simulink model "pv_model"  (R2023b)
settings: Solver=VariableStepAuto  StartTime=0.0  StopTime=10.0  RelTol=1e-3
libraries: simulink x1
settings Model: Creator=User  LastModifiedBy=User

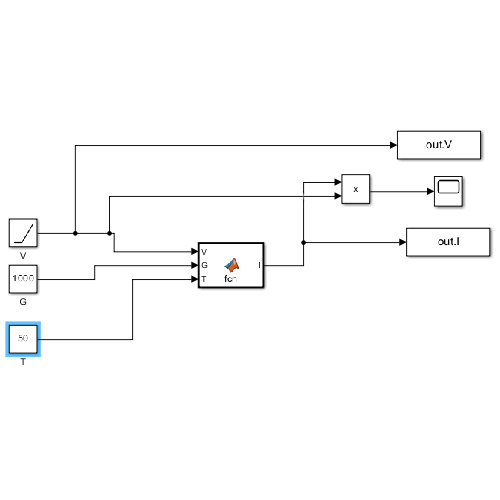
[thumbnail: Simulink's stored preview of the top-level diagram]
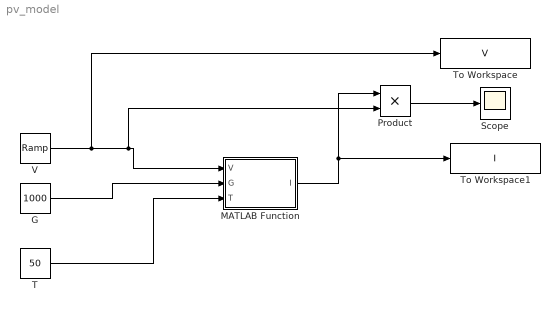
== system pv_model ==
  G : Constant  Value=1000
  MATLAB Function : MATLAB Function  TreatAsAtomicUnit=on
  Product : Product
  Scope : Scope
  T : Constant  Value=50
  To Workspace : ToWorkspace  VariableName=V  SaveFormat=Timeseries  SampleTime=-1
  To Workspace1 : ToWorkspace  VariableName=I  SaveFormat=Timeseries  SampleTime=-1
  V : simulink/Sources/Ramp  slope=3.76  start=0  InitialOutput=0
  wires:
  MATLAB Function/1(I) -> To Workspace1/1, Product/1
  V/1 -> To Workspace/1, Product/2, MATLAB Function/1(V)
  G/1 -> MATLAB Function/2(G)
  T/1 -> MATLAB Function/3(T)
  Product/1 -> Scope/1

== matlab function pv_model/MATLAB Function ==
  data: V input; I output; G input; T input
function I = fcn(V, G, T)
I = pv_model_func(V, G, T);

    
%     % Parametri panou (valori exemplu - ajustați cu datele reale)
%     persistent I_sc V_oc N_s k q n R_s R_p
%     if isempty(I_sc)
%         I_sc = 8.75;     % [A]
%         V_oc = 37.6;     % [V]
%         N_s = 60;        % Număr celule
%         k = 1.3806e-23;  % [J/K]
%         q = 1.6022e-19;  % [C]
%         n = 1.3;         % Factor idealitate
%         R_s = 0.2;       % [Ω]
%         R_p = 100;       % [Ω]
%     end
% 
%     % Calcule intermediare
%     I_ph = (G / 1000) * I_sc;
%     V_T = (k * (T + 273.15)) / q;
%     I_0 = I_sc / (exp(V_oc / (n * N_s * V_T)) - 1);
% 
%     % Rezolvare ecuație folosind metoda Newton-Raphson (mai stabilă decât fsolve)
%     I = I_ph; % Valoare inițială
%     for iter = 1:20
%         f = I - I_ph + I_0*(exp((V+I*R_s)/(n*N_s*V_T))-1) + (V+I*R_s)/R_p;
%         df = 1 + I_0*exp((V+I*R_s)/(n*N_s*V_T))*(R_s/(n*N_s*V_T)) + R_s/R_p;
%         I = I - f/df;
%     end
% end
